simulink model "adapted_control"  (R2018a)
settings: Solver=VariableStepAuto  StartTime=0.0  StopTime=10.0  RelTol=1e-3
libraries: neural x1
settings Model: Creator=ABHISHEK  LastModifiedBy=ABHISHEK

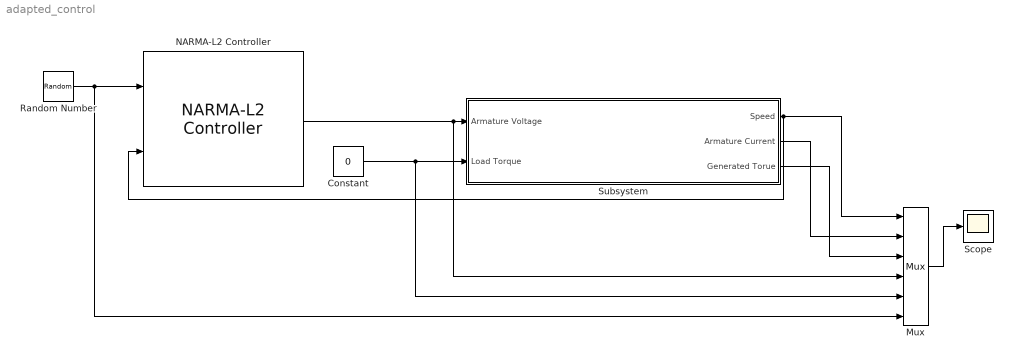
== system adapted_control ==
  Constant : Constant  Value=0
  Mux : Mux  Inputs=6
  NARMA-L2 Controller : neural/Control Systems/NARMA-L2 Controller  Normalize=0  IW1_1=[6.2058048238983403166 -1.5022478150954172715 -8.1675140530699117392 3.6488529633264099594;22.50046197409944071 1.5894035873031435724 -30.50439485418530694 12.773984985451821927;-3.3085139893802439914 -4.7529835331854917158 -9.272720115680000319 -1.5470291552214883168;-5.1353552915324849337 10.65225496005407102 -6.8505386127345211378 -3.6903864442581109095;-8.2466806469825133519 13.389133945129280789 -2.2372759460174727053 -5.6904552043979315101;0.19276749599107162458 -0.024017970983920167161 -1.3146868695421734226e-05 -0.33998362176119290012;1.0933378050767532663 1.951262720844163745 -4.7270429820206354421 0.47944914274779748542;0.41017704059778870018 6.3101108960456642194 -6.3935655425609363434 -0.22874695066198116877;23.240926740811680418 -67.673324336609226748 45.138209499808809255 18.101675238362421538;1.4147520893596743363 3.8427151870801123934 -4.2116784386011865138 0.53148068892845168332]  IW3_2=[2.1651899940207361972 0.23412494321297924738 -1.147218867803545761 -3.2112717487310282749;2.71702049296039716 -0.3372116625053789285 0.0018110214495279887328 -4.7597388136266056691;-0.47033996337266514853 -0.68518257915266755909 0.4517418647246752017 -0.33167269530489268403;-0.16709116556387351715 0.055085772835326618502 0.49841805812986400559 0.36784211037232655839;-2.2770861452049357965 0.6365023505886970856 2.8193926339365118494 -1.1593091849275647398;0.090090266985887346163 -0.016197928448296126241 -0.00047848026448624376462 -0.20839841468015676829;-0.16498680204521942727 0.017633344282655005753 0.0015239935164366958872 0.26947046967614035617;5.7729312553639697825 -0.7740444058789813786 0.19012677746706208026 -13.948619534274094178;-0.9476729607683280765 2.1004826813526706886 -0.75496721197843286166 -0.73137110494968304852;-0.34920569651623933893 0.42665940796768642151 0.0028697154653692263405 -0.24269560798407577296]  IW5_3=-0.3702808569782784498  LW2_1=[-0.23932529730531179601 0.011368191302672086759 0.279397528196487277 -0.011431991879333395015 -0.29817008616079565542 72.134651387570528414 0.13780446025020229306 0.12158735675239823459 -0.022439101674722197743 -0.12207112373157694152]  LW4_3=[0.0038329783422514540799 4.390027656272052603 -0.0016509638710626038573 0.0208771060989284378 0.0046790338928135513652 0.010144628067646290631 -0.048231428591223944602 -0.059199628315096619602 -0.0063840307459183615393 -0.0010388967495133893774]  LW5_4=0.81786694052308939185  LW6_5=-0.76030652324173420009  LW6_2=-0.91783932673275914205  B1=[2.0497987473210765863;39.15736432543094736;9.3363460236411217608;6.6936699581809611104;-2.2475518305823856124;0.44193568449886500016;-2.6464567030026904249;3.8432250318693035318;45.38297371142758152;-13.695933683163346473]  B2=-30.432127420110589355  B3=[2.4960192941992618287;6.9806347924551337414;-10.603333531963356151;2.815404655794206068;-5.9216971986859094912;6.9922047936464295503;5.1410445069065806578;-0.84231104751341290271;0.20082182645475735172;9.6106222996654793178]  B4=3.1604123437301128163  Limit_output=0  min_output=-Inf  max_output=Inf  Use_Previous_Weights=1  Ts=0.1  S1=10  Ni=2  Nj=3  sim_file=refmotor_model  trainfun=trainlm  Use_validation=1  Use_Testing=1  max_i=240  min_i=0  max_i_int=5  min_i_int=0.5  sam_training=1000  epochs=10  minp=0.078263121628543430575  maxp=239.55924625778359882  mint=0  maxt=239.55924625778359882
      settings: SourceProductName=Neural Network Toolbox  SourceProductBaseCode=NN
  Random Number : RandomNumber  Mean=120  Variance=200  SampleTime=1
  Scope : Scope
  Subsystem : Subsystem
  wires:
  Constant/1 -> Subsystem/2("Load Torque "), Mux/5
  NARMA-L2 Controller/1 -> Mux/4, Subsystem/1("Armature Voltage ")
  Subsystem/3("Generated Torue ") -> Mux/3
  Mux/1 -> Scope/1
  Subsystem/2(Armature Current) -> Mux/2
  Subsystem/1("Speed ") -> NARMA-L2 Controller/2, Mux/1
  Random Number/1 -> NARMA-L2 Controller/1, Mux/6

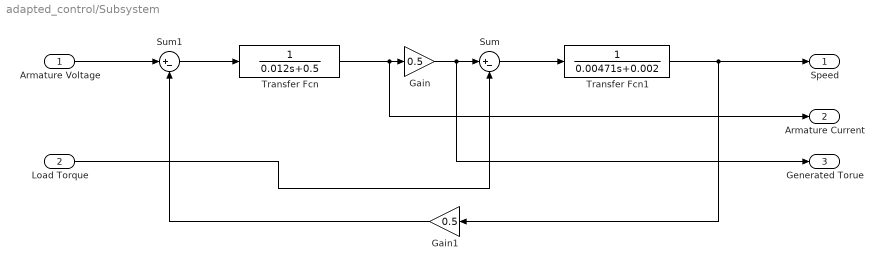
== system adapted_control/Subsystem ==
  "Armature Voltage " : Inport
  "Load Torque " : Inport  Port=2
  Gain : Gain  Gain=0.5
  Gain1 : Gain  Gain=0.5
  Sum : Sum  Inputs=|+-
  Sum1 : Sum  Inputs=|+-
  Transfer Fcn : TransferFcn  Denominator=[0.012 0.5]
  Transfer Fcn1 : TransferFcn  Denominator=[0.00471 0.002]
  "Speed " : Outport
  Armature Current : Outport  Port=2
  "Generated Torue " : Outport  Port=3
  wires:
  Gain1/1 -> Sum1/2
  Transfer Fcn/1 -> Armature Current/1, Gain/1
  Transfer Fcn1/1 -> "Speed "/1, Gain1/1
  "Armature Voltage "/1 -> Sum1/1
  Sum1/1 -> Transfer Fcn/1
  Gain/1 -> "Generated Torue "/1, Sum/1
  Sum/1 -> Transfer Fcn1/1
  "Load Torque "/1 -> Sum/2
